simulink model "UDP_Model"  (R2019a)
settings: Solver=VariableStepAuto  StartTime=0.0  StopTime=inf  RelTol=1e-3
undefined symbols (not defined in the file): f
libraries: aerolibconvert2 x3, xpcutilitieslib x2, instrumentlib x2
settings Model: Creator=10291  LastModifiedBy=10291

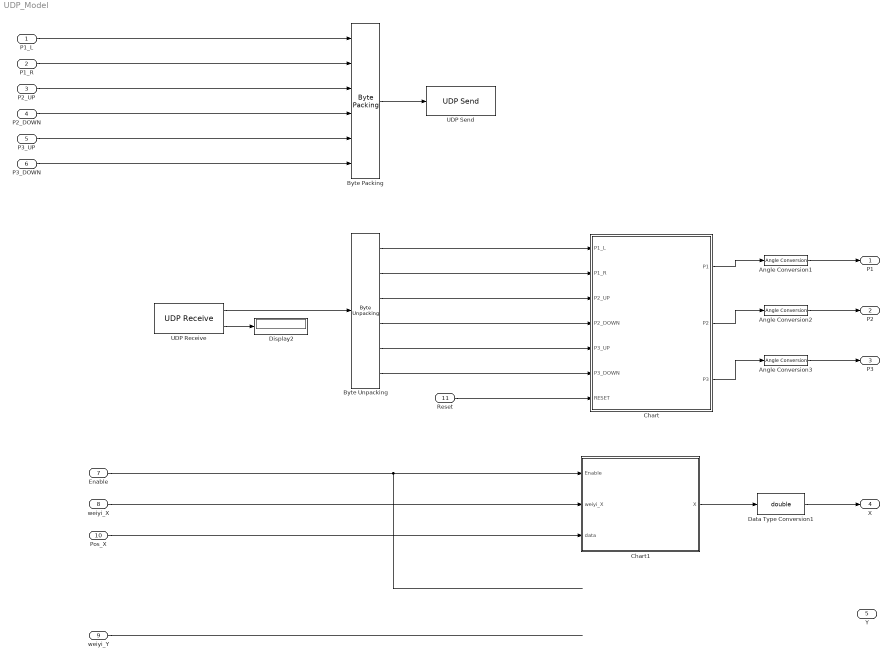
== system UDP_Model ==
  P1_L : Inport
  P1_R : Inport  Port=2
  P2_UP : Inport  Port=3
  P2_DOWN : Inport  Port=4
  P3_UP : Inport  Port=5
  P3_DOWN : Inport  Port=6
  Enable : Inport  Port=7  OutDataTypeStr=double
  weiyi_X : Inport  Port=8
  weiyi_Y : Inport  Port=9
  Pos_X : Inport  Port=10
  Reset : Inport  Port=11
  Angle Conversion1 : aerolibconvert2/Angle Conversion  IU=deg  OU=rad
  Angle Conversion2 : aerolibconvert2/Angle Conversion  IU=deg  OU=rad
  Angle Conversion3 : aerolibconvert2/Angle Conversion  IU=deg  OU=rad
  "Byte Packing " : xpcutilitieslib/Byte Packing   MaskPackedDataType=double  MaskUnpackedDataTypes={'uint8','uint8','uint8','uint8','uint8','uint8'}  MaskAlignment=1
  "Byte Unpacking " : xpcutilitieslib/Byte Unpacking   MaskUnpackedDataTypes={'uint8','uint8','uint8','uint8','uint8','uint8'}  MaskUnpackedDataSizes={[1],[1],[1],[1],[1],[1]}  MaskAlignment=1
      settings: SourceProductName=Simulink Real-Time  SourceProductBaseCode=XP
  Chart : Stateflow chart  TreatAsAtomicUnit=on
  Chart1 : Stateflow chart  BlockKeywords=__PRM__SERIALIZED__DATA__:Stateflow Chart,Stateflow Diagram  TreatAsAtomicUnit=on
  Data Type Conversion1 : DataTypeConversion  OutDataTypeStr=double
  Display2 : Display
  UDP Receive : instrumentlib/UDP Receive  Priority=3  Host=localhost  Port=51000  LocalPort=51001  EnablePortSharing=off  GetLatestData=off  DataSize=[1 1]  DataType=double  ASCIIFormatting=%f,  Terminator=LF  ByteOrder=BigEndian  EnableBlockingMode=off  Timeout=5  SampleTime=0.1  LocalAddress=0.0.0.0
      settings: SourceProductName=Instrument Control Toolbox
  UDP Send : instrumentlib/UDP Send  Priority=2  Host=localhost  Port=51001  LocalPort=51000  EnablePortSharing=off  ByteOrder=BigEndian  OutputDatagramPacketSize=10  EnableBlockingMode=on  LocalAddress=0.0.0.0
      settings: SourceProductName=Instrument Control Toolbox
  P1 : Outport
  P2 : Outport  Port=2
  P3 : Outport  Port=3
  X : Outport  Port=4
  Y : Outport  Port=5
  wires:
  "Byte Packing "/1 -> UDP Send/1
  UDP Receive/1 -> "Byte Unpacking "/1
  UDP Receive/2 -> Display2/1
  Chart/3(P3) -> Angle Conversion3/1
  Chart/2(P2) -> Angle Conversion2/1
  Chart/1(P1) -> Angle Conversion1/1
  Angle Conversion2/1 -> P2/1
  Angle Conversion3/1 -> P3/1
  Angle Conversion1/1 -> P1/1
  P1_L/1 -> "Byte Packing "/1
  P1_R/1 -> "Byte Packing "/2
  P2_UP/1 -> "Byte Packing "/3
  weiyi_X/1 -> Chart1/2(weiyi_X)
  Chart1/1(X) -> Data Type Conversion1/1
  ? -> Y/1
  weiyi_Y/1 -> ?
  Pos_X/1 -> Chart1/3(data)
  "Byte Unpacking "/1 -> Chart/1(P1_L)
  "Byte Unpacking "/2 -> Chart/2(P1_R)
  "Byte Unpacking "/3 -> Chart/3(P2_UP)
  "Byte Unpacking "/4 -> Chart/4(P2_DOWN)
  "Byte Unpacking "/5 -> Chart/5(P3_UP)
  "Byte Unpacking "/6 -> Chart/6(P3_DOWN)
  P2_DOWN/1 -> "Byte Packing "/4
  P3_UP/1 -> "Byte Packing "/5
  P3_DOWN/1 -> "Byte Packing "/6
  Reset/1 -> Chart/7(RESET)
  Enable/1 -> Chart1/1(Enable)
  Data Type Conversion1/1 -> X/1

== stateflow chart UDP_Model/Chart1 ==
  state a
    state zheng
      en:
      X = - pi * weiyi_X;
      Cnt = 0;
      du:
      Cnt = Cnt + 1;
    state fan
      en:
      Cnt = 0;
      du:
      X = pi * weiyi_X;
      Cnt = Cnt + 1;
    (default) -> zheng
    zheng -> fan : [after(1,sec)]
    fan -> zheng [order 2] : [after(1,sec)]
    fan -> (junction 31) [order 1] : [weiyi_X ~= 1]
  state aa
    state ss
      en:
      Cnt = 0;
      X = 45 * pi * Enable;
      du:
      Cnt = Cnt + 1;
    state ss1
      en:
      X = 0;
    ss -> ss1 : [after(1,sec)]
    (default) -> ss1
  aa -> a : [weiyi_X == 1]
  (default) -> aa
  (junction 31) -> ss
  data: X output double; Enable input; weiyi_X input; data input; Cnt local uint8

== stateflow chart UDP_Model/Chart ==
  state b
    b -> (junction 75) [order 1]
    (junction 75) -> (junction 88) [order 1] : [P1_L == 1]
    (junction 75) -> (junction 90) [order 2]
    (junction 88) -> (junction 84) : {P1 = P1 + 0.1;}
    (junction 84) -> (junction 90)
    (junction 90) -> (junction 86)
    (junction 86) -> (junction 85) [order 1] : [P1_R == 1]
    (junction 86) -> (junction 91) [order 2]
    (junction 85) -> (junction 87) : {P1 = P1 - 0.1;}
    (junction 87) -> (junction 91)
    (junction 91) -> (junction 74)
    (junction 74) -> (junction 98) [order 1] : [P2_UP == 1]
    (junction 74) -> (junction 106) [order 2]
    (junction 98) -> (junction 104) : {P2 = P2 + 0.1;}
    (junction 104) -> (junction 106)
    (junction 106) -> (junction 100)
    (junction 100) -> (junction 101) [order 1] : [P2_DOWN == 1]
    (junction 100) -> (junction 112) [order 2]
    (junction 101) -> (junction 110) : {P2 = P2 - 0.1;}
    (junction 110) -> (junction 112)
    (junction 112) -> (junction 131)
    (junction 131) -> (junction 127) [order 1] : [P3_UP == 1]
    (junction 131) -> (junction 123) [order 2]
    (junction 127) -> (junction 117) : {P3 = P3 + 0.1;}
    (junction 117) -> (junction 123)
    (junction 123) -> (junction 128)
    (junction 128) -> (junction 119) [order 1] : [P3_DOWN == 1]
    (junction 128) -> (junction 115) [order 2]
    (junction 119) -> (junction 124) : {P3 = P3 - 0.1;}
    (junction 124) -> (junction 115)
    (junction 115) -> (junction 133)
  state a
    en:
    P1 = 0;
    P2 = 0;
    P3 = 180;
  (default) -> a
  a -> b : [after(1,tick)]
  b -> a [order 1] : [RESET == 1]
  data: P1 output; P2 output double; P3 output double; P1_L input; P1_R input; P2_UP input; P2_DOWN input; P3_UP input; P3_DOWN input; RESET input
